simulink model "buck_lsm"  (R2021a)
settings: Solver=ode23tb  StartTime=0.0  StopTime=0.5  RelTol=1e-3
values from neighbouring files (symbols this model uses):
  C = ( irip * Ts ) / (8 * vrip)    (= 5.20833333333e-06)    [lsm.m]
  D = (V)/(Vg-(Iout*Rg))    (= 0.447204968944)    [lsm.m]
  L = ((Vg - V) / (2*irip)) * D * Ts    (= 8.58633540373e-05)    [lsm.m]
  Rg = 140e-3    (= 0.14)    [lsm.m]
  Rl = V/Iout    (= 1.44)    [lsm.m]
  Vg = 28    [lsm.m]
libraries: spsSeriesRLCBranchLib x8, spsControlledVoltageSourceLib x5, spsGroundLib x4, spsCurrentMeasurementLib x3, spsVoltageMeasurementLib x3, spsControlledCurrentSourceLib x2, spsDCVoltageSourceLib x2, spsIdealSwitchLib x2, spsPWMGeneratorDCDCLib x1, spspowerguiLib x1
settings Model: Creator=yoshi  LastModifiedBy=yoshi

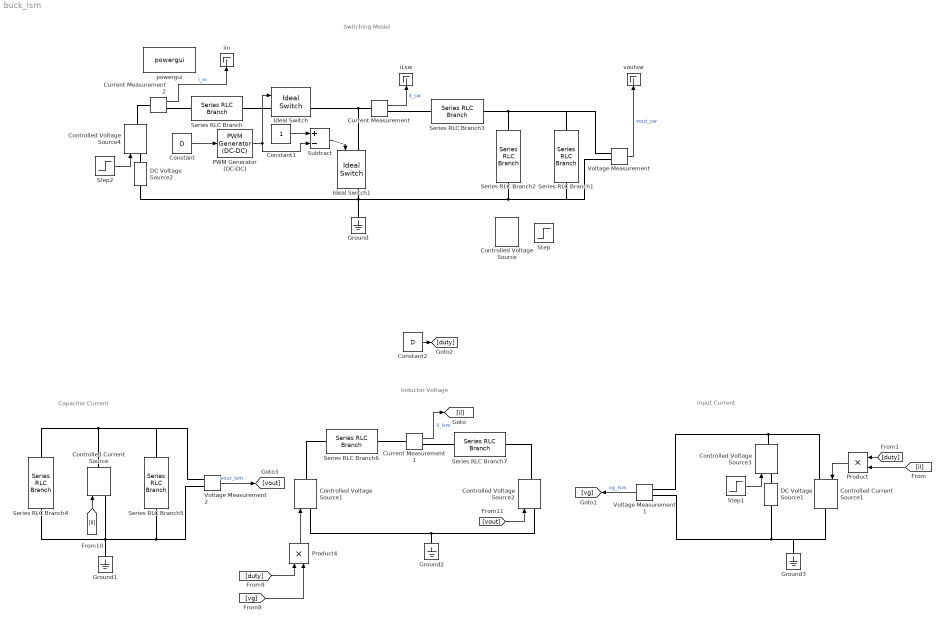
== system buck_lsm ==
  note: Inductor Voltage
  note: Capacitor Current
  note: Input Current
  note: Switching Model
  Constant : Constant  Value=D
  Constant1 : Constant
  Constant2 : Constant  Value=D
  Controlled Current Source : spsControlledCurrentSourceLib/Controlled Current Source  Initialize=on  Source_Type=AC  Amplitude=0  Phase=0  Frequency=0  Measurements=None
  Controlled Current Source1 : spsControlledCurrentSourceLib/Controlled Current Source  Initialize=on  Source_Type=AC  Amplitude=0  Phase=0  Frequency=0  Measurements=None
  Controlled Voltage Source : spsControlledVoltageSourceLib/Controlled Voltage Source  Initialize=on  Source_Type=DC  Amplitude=0  Phase=0  Frequency=0  Measurements=None
  Controlled Voltage Source1 : spsControlledVoltageSourceLib/Controlled Voltage Source  Initialize=on  Source_Type=AC  Amplitude=0  Phase=0  Frequency=0  Measurements=None
  Controlled Voltage Source2 : spsControlledVoltageSourceLib/Controlled Voltage Source  Initialize=on  Source_Type=AC  Amplitude=0  Phase=0  Frequency=0  Measurements=None
  Controlled Voltage Source3 : spsControlledVoltageSourceLib/Controlled Voltage Source  Initialize=on  Source_Type=DC  Amplitude=0  Phase=0  Frequency=0  Measurements=None
  Controlled Voltage Source4 : spsControlledVoltageSourceLib/Controlled Voltage Source  Initialize=on  Source_Type=DC  Amplitude=6  Phase=0  Frequency=0  Measurements=None
  Current Measurement : spsCurrentMeasurementLib/Current Measurement  PhasorSimulation=off  OutputType=Complex  PSBequivalent=0
  Current Measurement1 : spsCurrentMeasurementLib/Current Measurement  PhasorSimulation=off  OutputType=Complex  PSBequivalent=0
  Current Measurement2 : spsCurrentMeasurementLib/Current Measurement  PhasorSimulation=off  OutputType=Complex  PSBequivalent=0
  DC Voltage Source1 : spsDCVoltageSourceLib/DC Voltage Source  Amplitude=Vg  Measurements=None
  DC Voltage Source2 : spsDCVoltageSourceLib/DC Voltage Source  Amplitude=Vg  Measurements=None
  Ground{,1..3} (4 alike) : spsGroundLib/Ground  LConnTagsString=a
  Ideal Switch : spsIdealSwitchLib/Ideal Switch  Ron=0.001  Lon=0  IC=0  Rs=1e5  Cs=inf  Measurements=on
  Ideal Switch1 : spsIdealSwitchLib/Ideal Switch  Ron=0.001  Lon=0  IC=0  Rs=1e5  Cs=inf  Measurements=on
  PWM Generator (DC-DC) : spsPWMGeneratorDCDCLib/PWM Generator (DC-DC)  Fsw=fsw  Ts=0
  Product : Product
  Product4 : Product
  Series RLC Branch : spsSeriesRLCBranchLib/Series RLC Branch  LConnTagsString=__new0  RConnTagsString=__new0  BranchType=R  Resistance=Rg  Inductance=1e-3  SetiL0=off  InitialCurrent=0  Capacitance=1e-6  Setx0=off  InitialVoltage=0  Measurements=None
  Series RLC Branch1 : spsSeriesRLCBranchLib/Series RLC Branch  LConnTagsString=__new0  RConnTagsString=__new0  BranchType=R  Resistance=Rl  Inductance=1e-3  SetiL0=off  InitialCurrent=0  Capacitance=1e-6  Setx0=off  InitialVoltage=0  Measurements=None
  Series RLC Branch2 : spsSeriesRLCBranchLib/Series RLC Branch  LConnTagsString=__new0  RConnTagsString=__new0  BranchType=C  Resistance=1  Inductance=1e-3  SetiL0=off  InitialCurrent=0  Capacitance=C  Setx0=off  InitialVoltage=0  Measurements=None
  Series RLC Branch3 : spsSeriesRLCBranchLib/Series RLC Branch  LConnTagsString=__new0  RConnTagsString=__new0  BranchType=L  Resistance=1  Inductance=L  SetiL0=off  InitialCurrent=0  Capacitance=1e-6  Setx0=off  InitialVoltage=0  Measurements=None
  Series RLC Branch4 : spsSeriesRLCBranchLib/Series RLC Branch  LConnTagsString=__new0  RConnTagsString=__new0  BranchType=C  Resistance=1  Inductance=1e-3  SetiL0=off  InitialCurrent=0  Capacitance=C  Setx0=off  InitialVoltage=0  Measurements=None
  Series RLC Branch5 : spsSeriesRLCBranchLib/Series RLC Branch  LConnTagsString=__new0  RConnTagsString=__new0  BranchType=R  Resistance=Rl  Inductance=1e-3  SetiL0=off  InitialCurrent=0  Capacitance=1e-6  Setx0=off  InitialVoltage=0  Measurements=None
  Series RLC Branch6 : spsSeriesRLCBranchLib/Series RLC Branch  LConnTagsString=__new0  RConnTagsString=__new0  BranchType=R  Resistance=Rg  Inductance=1e-3  SetiL0=off  InitialCurrent=0  Capacitance=1e-6  Setx0=off  InitialVoltage=0  Measurements=None
  Series RLC Branch7 : spsSeriesRLCBranchLib/Series RLC Branch  LConnTagsString=__new0  RConnTagsString=__new0  BranchType=L  Resistance=1  Inductance=L  SetiL0=off  InitialCurrent=0  Capacitance=1e-6  Setx0=off  InitialVoltage=0  Measurements=None
  Step : Step  SampleTime=0
  Step1 : Step  Time=0.002  After=6  SampleTime=0
  Step2 : Step  Time=0.002  After=6  SampleTime=0
  Subtract : Sum  Inputs=+-
  Voltage Measurement : spsVoltageMeasurementLib/Voltage Measurement  PhasorSimulation=off  OutputType=Complex  PSBequivalent=0
  Voltage Measurement1 : spsVoltageMeasurementLib/Voltage Measurement  PhasorSimulation=off  OutputType=Complex  PSBequivalent=0
  Voltage Measurement2 : spsVoltageMeasurementLib/Voltage Measurement  PhasorSimulation=off  OutputType=Complex  PSBequivalent=0
  iLsw : Terminator
  iin : Terminator
  powergui : spspowerguiLib/powergui  Priority=1  SimulationMode=Continuous  SampleTime=50e-6  frequency=60  Iterations=50  frequencyindice=0  Pbase=100e6  ErrMax=1e-4  UnitsV=kV  UnitsW=MW  buscounter=0  FunctionMessages=off  echomessages=off  EnableUseOfTLC=off  CurrentSourceSwitches=off  DisableSnubberDevices=off  DisableRonSwitches=off  DisableVfSwitches=off  DisplayEquations=off  AutomaticDiscreteSolvers=off  SolverType=Tustin/Backward Euler (TBE)  Interpol=off  ExternalGateDelay=off  methode=off  Ts=100  x0status=blocks  SPID=on  SwTol=0  HookPort=off  NonlinearTolerance=1e-4  nMaxIteration=100  ContinueOnMaxIteration=off  RestoreLinks=warning  ResistiveCurrentMeasurement=off  Frange=[0:2:500]  Ylog=off  Xlog=on  ShowGrid=off  save=off  variable=ZData  structure=0  ZoomFFT=off  StartTime=0.0  cycles=1  DisplayStyle=1  fundamental=60  FreqAxis=off  MaxFrequency=1000  frequencyindicesteady=1  RmsSteady=1  display=off
  voutsw : Terminator
  wires:
  PWM Generator (DC-DC)/1 -> Subtract/2, Ideal Switch/1
  Constant/1 -> PWM Generator (DC-DC)/1
  Current Measurement/1 -> iLsw/1  "il_sw"
  Voltage Measurement/1 -> voutsw/1  "vout_sw"
  Subtract/1 -> Ideal Switch1/1
  Constant1/1 -> Subtract/1
  Current Measurement1/1 -> [il]  "il_lsm"
  Voltage Measurement1/1 -> [vg]  "vg_lsm"
  Constant2/1 -> [duty]
  [il] -> Product/2
  [duty] -> Product/1
  Product/1 -> Controlled Current Source1/1
  [vg] -> Product4/2
  [duty] -> Product4/1
  Product4/1 -> Controlled Voltage Source1/1
  [il] -> Controlled Current Source/1
  Voltage Measurement2/1 -> [vout]  "vout_lsm"
  [vout] -> Controlled Voltage Source2/1
  Step1/1 -> Controlled Voltage Source3/1
  Step2/1 -> Controlled Voltage Source4/1
  Current Measurement2/1 -> iin/1  "i_in"
  connections:
  Ground/LConn1 -- DC Voltage Source2/LConn1 -- Voltage Measurement/LConn2 -- Series RLC Branch1/RConn1 -- Series RLC Branch2/RConn1 -- Ideal Switch1/RConn1
  Ideal Switch1/LConn1 -- Ideal Switch/RConn1 -- Current Measurement/LConn1
  Ideal Switch/LConn1 -- Series RLC Branch/RConn1
  Series RLC Branch2/LConn1 -- Voltage Measurement/LConn1 -- Series RLC Branch1/LConn1 -- Series RLC Branch3/RConn1
  Current Measurement/RConn1 -- Series RLC Branch3/LConn1
  Controlled Current Source/RConn1 -- Series RLC Branch5/LConn1 -- Voltage Measurement2/LConn1 -- Series RLC Branch4/LConn1
  Series RLC Branch4/RConn1 -- Ground1/LConn1 -- Controlled Current Source/LConn1 -- Voltage Measurement2/LConn2 -- Series RLC Branch5/RConn1
  Series RLC Branch6/RConn1 -- Current Measurement1/LConn1
  Voltage Measurement1/LConn1 -- Controlled Voltage Source3/RConn1 -- Controlled Current Source1/LConn1
  Voltage Measurement1/LConn2 -- Controlled Current Source1/RConn1 -- Ground3/LConn1 -- DC Voltage Source1/LConn1
  Controlled Voltage Source1/RConn1 -- Series RLC Branch6/LConn1
  Series RLC Branch7/RConn1 -- Controlled Voltage Source2/RConn1
  Controlled Voltage Source2/LConn1 -- Ground2/LConn1 -- Controlled Voltage Source1/LConn1
  Current Measurement1/RConn1 -- Series RLC Branch7/LConn1
  Controlled Voltage Source3/LConn1 -- DC Voltage Source1/RConn1
  Controlled Voltage Source4/LConn1 -- DC Voltage Source2/RConn1
  Current Measurement2/RConn1 -- Series RLC Branch/LConn1
  Current Measurement2/LConn1 -- Controlled Voltage Source4/RConn1
